simulink model "SS_task6_5"  (R2021b)
settings: Solver=FixedStepAuto  StartTime=0.0  StopTime=10.0  FixedStep=0.01  RelTol=1e-3
values from neighbouring files (symbols this model uses):
  A_ss = [ 0 1 0 0 ... (first row only)    [Copy_of_Lab_3_ale.m]    (also in Lab_3_ale.m; mass_2dof.m)
  B_ss = [0 0 0 ... (first row only)    [Copy_of_Lab_3_ale.m]    (also in Lab_3_ale.m = [0 0; mass_2dof.m)
  C_ss = [1 0 0 0]    [Copy_of_Lab_3_ale.m]    (also in Lab_3_ale.m; mass_2dof.m)
  D_ss = [0 0 0]    [Copy_of_Lab_3_ale.m]    (also in Lab_3_ale.m = [0 0]; mass_2dof.m)
  wn = wn_und_1dof    [Copy_of_Lab_3_ale.m]    (also in H_inf_ctrl_11_2.m = eig(Ask); H_inf_ctrl_11_2_m.m = eig(Ask); Lab_3_ale.m = sqrt(kp/mp); mass_2dof.m)
undefined symbols (not defined in the file or in its folder): sigbuilder_block
settings Model: Creator=rivaa  LastModifiedBy=rivaa

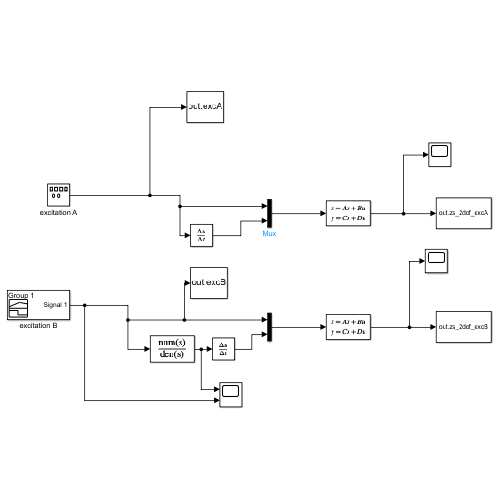
[thumbnail: Simulink's stored preview of the top-level diagram]
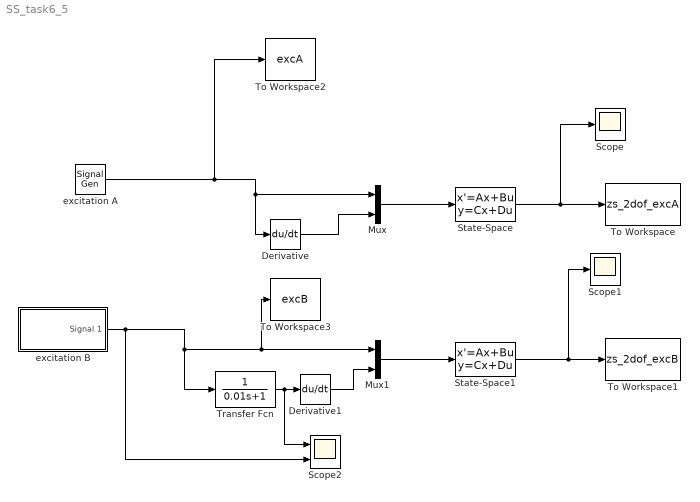
== system SS_task6_5 ==
  Derivative : Derivative
  Derivative1 : Derivative
  Mux : Mux  Inputs=2
  Mux1 : Mux  Inputs=2
  Scope : Scope
  Scope1 : Scope
  Scope2 : Scope  NumInputPorts=2
  State-Space : StateSpace  A=A_ss  B=B_ss  C=C_ss  D=D_ss  InitialCondition=0
  State-Space1 : StateSpace  A=A_ss  B=B_ss  C=C_ss  D=D_ss  InitialCondition=0
  To Workspace : ToWorkspace  VariableName=zs_2dof_excA  SampleTime=-1
      settings: Save2DSignal=2-D array (concatenate along first dimension)
  To Workspace1 : ToWorkspace  VariableName=zs_2dof_excB  SampleTime=-1
      settings: Save2DSignal=2-D array (concatenate along first dimension)
  To Workspace2 : ToWorkspace  VariableName=excA  SampleTime=-1
      settings: Save2DSignal=2-D array (concatenate along first dimension)
  To Workspace3 : ToWorkspace  VariableName=excB  SampleTime=-1
      settings: Save2DSignal=2-D array (concatenate along first dimension)
  Transfer Fcn : TransferFcn  Denominator=[0.01 1]
  excitation A : SignalGenerator  Amplitude=0.05  Frequency=wn  Units=rad/sec
  excitation B : Subsystem  Tag=STV Subsys  LoadFcn=sigbuilder_block('load');  StartFcn=sigbuilder_block('start');  StopFcn=sigbuilder_block('stop');  ClipboardFcn=sigbuilder_block('clipboard');  mask(Sigbuilder block){tuvar=[0:10]}
      mask help: Simulink:masks:SigbuilderBlock_MD
      mask init:
      | if ~strcmp(get_param(bdroot(gcbh),'SimulationStatus'),'stopped') tuvar = sigbuilder_block('maskInit'); end
      settings: CopyFcn=sigbuilder_block('copy');  DeleteFcn=sigbuilder_block('delete');  ModelCloseFcn=sigbuilder_block('modelClose');  PreSaveFcn=sigbuilder_block('preSave');  PauseFcn=sigbuilder_block('pause');  ContinueFcn=sigbuilder_block('continue');  NameChangeFcn=sigbuilder_block('namechange');  OpenFcn=sigbuilder_block('open',[437.6 199.2 550.4 400 ]);  CloseFcn=sigbuilder_block('close');
      mask Display: plot(0, 0, 100, 100,[2, 2, 32, 32, 2], [68, 8, 8, 68, 68],[32, 2], [38, 38], [32, 19, 2],[53, 60, 44], [32, 17, 17, 2],[16, 16, 31, 31]);txt = getActiveGroup(gcbh);text(2, 100, txt,'verticalAlignment', 'top');
  wires:
  State-Space/1 -> Scope/1, To Workspace/1
  excitation A/1 -> To Workspace2/1, Derivative/1, Mux/1
  Derivative/1 -> Mux/2
  Mux/1 -> State-Space/1
  Mux1/1 -> State-Space1/1
  Derivative1/1 -> Mux1/2
  excitation B/1(Signal 1) -> Scope2/2, To Workspace3/1, Mux1/1, Transfer Fcn/1
  State-Space1/1 -> Scope1/1, To Workspace1/1
  Transfer Fcn/1 -> Scope2/1, Derivative1/1

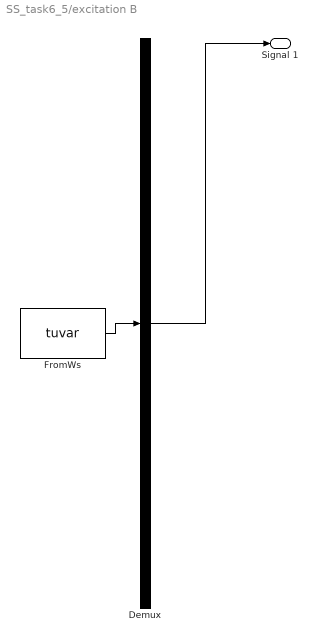
== system SS_task6_5/excitation B ==
  Demux : Demux  Tag=STV Demux  Outputs=1
      settings: DisplayOption=none
  FromWs : FromWorkspace  Tag=STV FromWs  VariableName=tuvar
      SigBuilderData=|
      | common.afterFinalStr = 'Extrapolate'
      | common.sampleTime = 0
      | dataSet.timeRange = [0 10]
      | dataSet.name = 'Group 1'
      | sbobj.Groups.Name = 'Group 1'
      | sbobj.Groups.Signals.Name = 'Signal 1'
      | sbobj.Groups.Signals.XData = [0 4 4 4.1 4.1 10]
      | sbobj.Groups.Signals.YData = [0 0 0.05 0.05 0 0]
  Signal 1 : Outport  Tag=STV Outport
  wires:
  Demux/1 -> Signal 1/1
  FromWs/1 -> Demux/1
